simulink model "Q3_Dynamic_vibration_abordes"  (R2024b)
settings: Solver=VariableStepAuto  StartTime=0.0  StopTime=t  RelTol=1e-3
model workspace (MAT data in the model file):
  K1 = 100
  K12 = 800
  M1 = 20
  M2 = 200
  b = 100
  t = 50
settings Model: Creator=chall  LastModifiedBy=chall

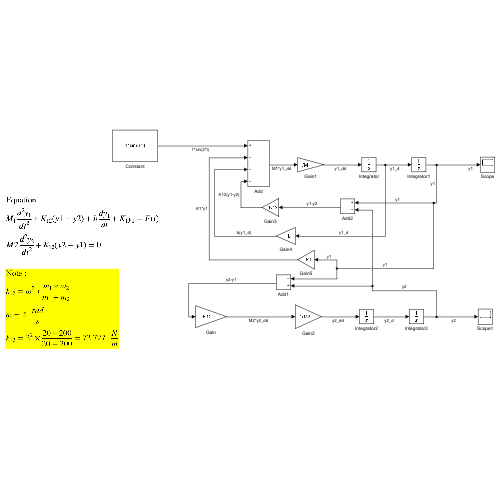
[thumbnail: Simulink's stored preview of the top-level diagram]
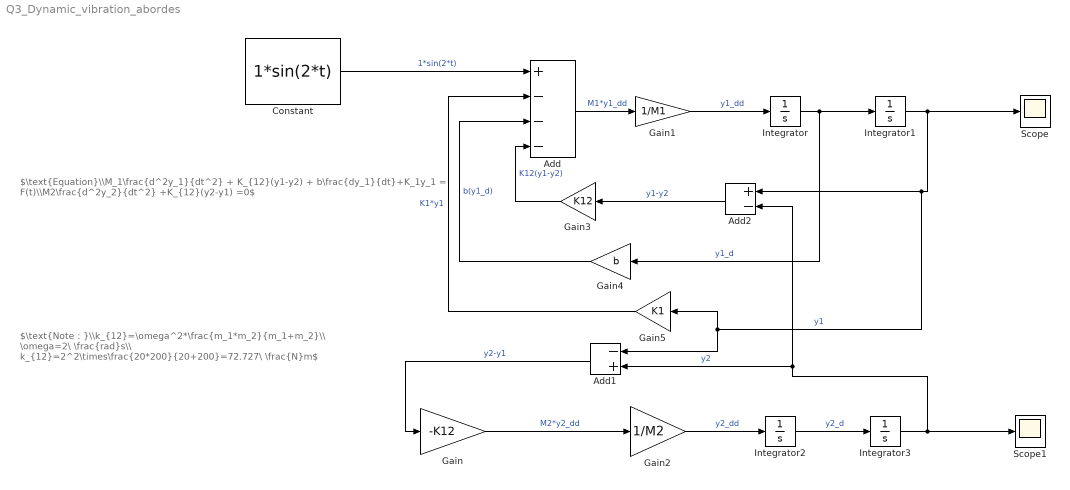
== system Q3_Dynamic_vibration_abordes ==
  note: $\text{Note : }\\k_{12}=\omega^2*\frac{m_1*m_2}{m_1+m_2}\\ \omega=2\ \frac{rad}s\\ k_{12}=2^2\times\frac{20*200}{20+200}=72.727\ \frac{N}m$
  note: $\text{Equation}\\M_1\frac{d^2y_1}{dt^2} + K_{12}(y1-y2) + b\frac{dy_1}{dt}+K_1y_1 = F(t)\\M2\frac{d^2y_2}{dt^2} +K_{12}(y2-y1) =0$
  Add : Sum  Inputs=+---
  Add1 : Sum  Inputs=-+
  Add2 : Sum  Inputs=+-
  Constant : Constant  Value=1*sin(2*t)
  Gain : Gain  Gain=-K12
  Gain1 : Gain  Gain=1/M1
  Gain2 : Gain  Gain=1/M2
  Gain3 : Gain  Gain=K12
  Gain4 : Gain  Gain=b
  Gain5 : Gain  Gain=K1
  Integrator{,1..3} (4 alike) : Integrator
  Scope : Scope
  Scope1 : Scope
  wires:
  Gain1/1 -> Integrator/1  "y1_dd"
  Integrator/1 -> Gain4/1, Integrator1/1  "y1_d"
  Integrator1/1 -> Scope/1, Add1/1, Gain5/1, Add2/1  "y1"
  Add/1 -> Gain1/1  "M1*y1_dd"
  Gain/1 -> Gain2/1  "M2*y2_dd"
  Gain2/1 -> Integrator2/1  "y2_dd"
  Integrator2/1 -> Integrator3/1  "y2_d"
  Integrator3/1 -> Add2/2, Add1/2, Scope1/1  "y2"
  Add1/1 -> Gain/1  "y2-y1"
  Add2/1 -> Gain3/1  "y1-y2"
  Gain3/1 -> Add/4  "K12(y1-y2)"
  Gain4/1 -> Add/3  "b(y1_d)"
  Gain5/1 -> Add/2  "K1*y1"
  Constant/1 -> Add/1  "1*sin(2*t)"
